simulink model "Simulation_ClosedLoop"  (R2018a)
settings: Solver=VariableStepAuto  StartTime=ti  StopTime=tf  RelTol=1e-3
StopFcn:
  | PlotTimeMotor;
undefined symbols (not defined in the file or in its folder): A_real, B_real, Cx_nominal, D_real, G, IC, K, Noise, thetac, torque, umax
libraries: simulink x1
settings Model: Creator=perruquetti  LastModifiedBy=perruquetti

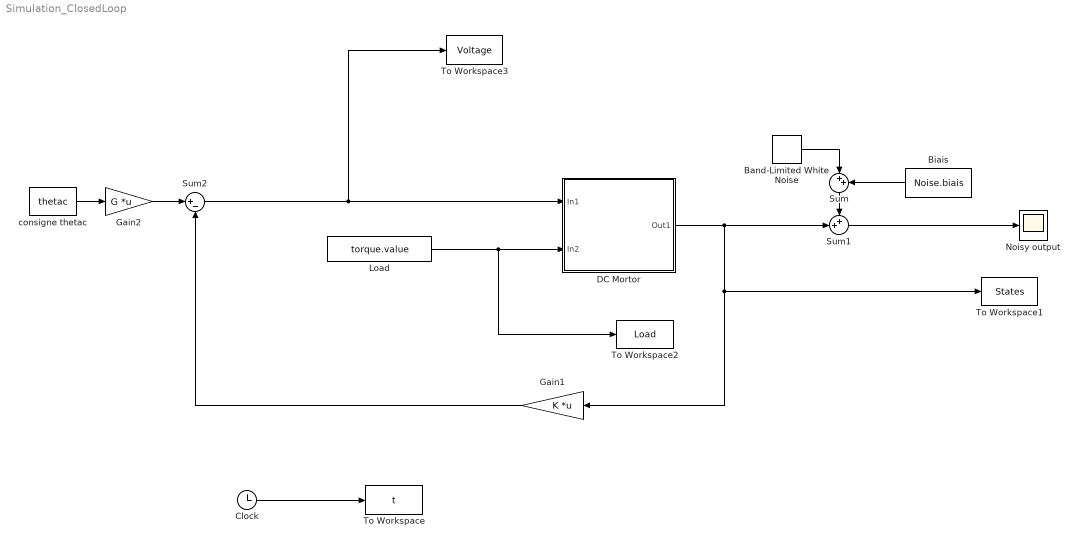
== system Simulation_ClosedLoop ==
  Band-Limited White Noise : simulink/Sources/Band-Limited White Noise  Cov=Noise.power  Ts=Noise.sampling  seed=Noise.seed
  Biais : Constant  Value=Noise.biais
  Clock : Clock
  DC Mortor : Subsystem
      mask Display: image('motor2.png');
  Gain1 : Gain  Gain=K  Multiplication=Matrix(K*u)
  Gain2 : Gain  Gain=G  Multiplication=Matrix(K*u)
  Load : Constant  Value=torque.value
  Noisy output : Scope
  Sum : Sum  Inputs=|++
  Sum1 : Sum  Inputs=++|
  Sum2 : Sum  Inputs=|+-
  To Workspace : ToWorkspace  VariableName=t  SampleTime=-1
  To Workspace1 : ToWorkspace  VariableName=States  SampleTime=-1
  To Workspace2 : ToWorkspace  VariableName=Load  SampleTime=-1
  To Workspace3 : ToWorkspace  VariableName=Voltage  SampleTime=-1
  consigne thetac : Constant  Value=thetac
  wires:
  Band-Limited White Noise/1 -> Sum/1
  Biais/1 -> Sum/2
  Sum/1 -> Sum1/1
  Sum1/1 -> Noisy output/1
  Clock/1 -> To Workspace/1
  DC Mortor/1(Out1) -> To Workspace1/1, Gain1/1, Sum1/2
  Sum2/1 -> To Workspace3/1, DC Mortor/1(In1)
  Load/1 -> To Workspace2/1, DC Mortor/2(In2)
  consigne thetac/1 -> Gain2/1
  Gain2/1 -> Sum2/1
  Gain1/1 -> Sum2/2

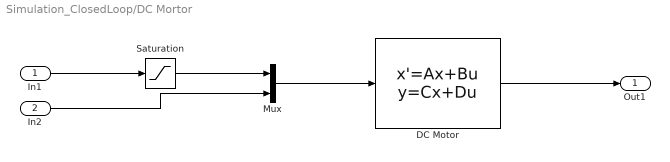
== system Simulation_ClosedLoop/DC Mortor ==
  In1 : Inport
  In2 : Inport  Port=2
  DC Motor : StateSpace  A=A_real  B=B_real  C=Cx_nominal  D=D_real  InitialCondition=IC.state
  Mux : Mux  Inputs=2
  Saturation : Saturate  UpperLimit=umax  LowerLimit=-umax
  Out1 : Outport
  wires:
  DC Motor/1 -> Out1/1
  In1/1 -> Saturation/1
  Saturation/1 -> Mux/1
  Mux/1 -> DC Motor/1
  In2/1 -> Mux/2
